simulink model "mainModel"  (R2018b)
settings: Solver=ode15s  StartTime=0.0  StopTime=sim_time  MaxStep=maxStep* tp.lengthScaleFactor^0.5
values from neighbouring files (symbols this model uses):
  grav = 9.81    [mainModel_ts.m]
  MI = [14330000 0 0; 0 143200 0; 0 0 15300000]    [mainModel_ts.m]
undefined symbols (not defined in the file or in its folder): env_t, tp
libraries: tethersNCsContrl_cl x1, fixedGroundStation_cl x1, avl2DLiftingBdy_cl x1, partitionedLifitngBdy_cls x1, kelvinVoigtTether_cl x1, pureIntegratorWinch_cl x1
settings Model: SimulationMode=accelerator  Creator=Ayaz  LastModifiedBy=asiddiq2

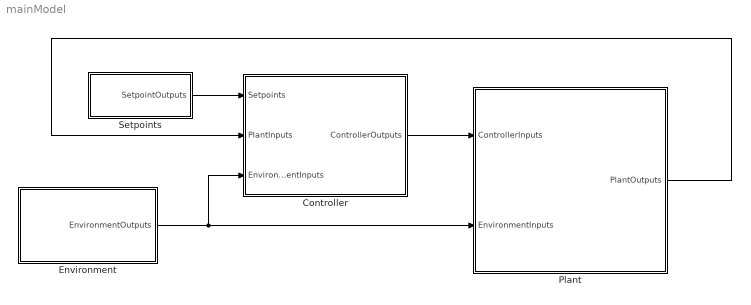
== system mainModel ==
  Controller : Subsystem
  Environment : Subsystem
  Plant : Subsystem
  Setpoints : Subsystem
  wires:
  Environment/1(EnvironmentOutputs) -> Plant/2(EnvironmentInputs), Controller/3(EnvironmentInputs)
  Plant/1(PlantOutputs) -> Controller/2(PlantInputs)
  Controller/1(ControllerOutputs) -> Plant/1(ControllerInputs)
  Setpoints/1(SetpointOutputs) -> Controller/1(Setpoints)

== system mainModel/Controller ==
  Setpoints : Inport
  PlantInputs : Inport  Port=2
  EnvironmentInputs : Inport  Port=3
  Variant Subsystem : Subsystem  VariantControlMode=Label  Variant=on  LabelModeActiveChoice=tethersNCsVariant  mask{ctlr_var=Simple Tether and Control Surfaces}
      mask prompts: ctlr_var "Choose Controller Variant"
      mask init:
      | choice = get_param(gcb,'ctlr_var');
      | vssBlk = gcb;
      | 
      | if strcmp(choice,'Simple Tether and Control Surfaces')
      |     set_param(vssBlk, 'OverrideUsingVariant', 'tethersNCsVariant');
      |     
      | elseif strcmp(choice,'No Controller')
      |     set_param(vssBlk, 'OverrideUsingVariant', 'NoControl');
      |     
      | end
      mask TypeOptions ctlr_var: Simple Tether and Control Surfaces | No Controller
  ControllerOutputs : Outport
  wires:
  EnvironmentInputs/1 -> Variant Subsystem/3(EnvironmentOutputs)
  PlantInputs/1 -> Variant Subsystem/2(PlantOutputs)
  Setpoints/1 -> Variant Subsystem/1(Setpoints)
  Variant Subsystem/1(ControllerOutputs) -> ControllerOutputs/1

== system mainModel/Environment ==
  Bus Creator : BusCreator  Inputs=1
  Constant : Constant  Value=env_t.inertialFlowVel.value  VectorParams1D=off
  Reshape : Reshape  OutputDimensionality=Column vector (2-D)
  EnvironmentOutputs : Outport
  wires:
  Constant/1 -> Reshape/1
  Reshape/1 -> Bus Creator/1  "inertialFlowVel"
  Bus Creator/1 -> EnvironmentOutputs/1

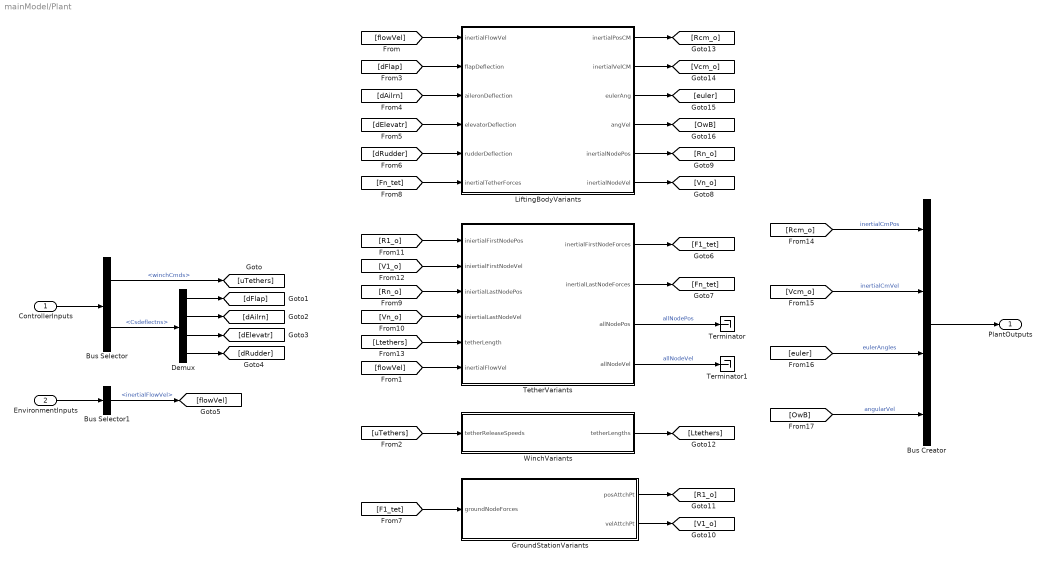
== system mainModel/Plant ==
  ControllerInputs : Inport
  EnvironmentInputs : Inport  Port=2
  Bus Creator : BusCreator  Inputs=4
  Bus Selector : BusSelector  OutputSignals=winchCmds,Csdeflectns
  Bus Selector1 : BusSelector  OutputSignals=inertialFlowVel
  Demux : Demux
  GroundStationVariants : Subsystem  VariantControlMode=Label  Variant=on  LabelModeActiveChoice=FixedVariant  mask{gndStatnMdl=Fixed Ground Station}
      mask prompts: gndStatnMdl "Choose Ground Station Model"
      mask init:
      | choice = get_param(gcb,'gndStatnMdl');
      | vssBlk = gcb;
      | 
      | if strcmp(choice,'Fixed Ground Station')
      |     set_param(vssBlk, 'OverrideUsingVariant', 'FixedVariant');
      |     
      | elseif strcmp(choice,'Floating Ground Station')
      |     set_param(vssBlk, 'OverrideUsingVariant', 'FloatingVariant');
      |     
      | end
      mask TypeOptions gndStatnMdl: Fixed Ground Station | Floating Ground Station
  LiftingBodyVariants : Subsystem  VariantControlMode=Label  Variant=on  LabelModeActiveChoice=partitionedLftingBdyVariant  mask{lftingbdyMdl=Partitioned Lifting Body}
      mask prompts: lftingbdyMdl "Choose Lifting Body Model"
      mask init:
      | choice = get_param(gcb,'lftingbdyMdl');
      | vssBlk = gcb;
      | 
      | if strcmp(choice,'AVL 2D Lifting Body')
      |     set_param(vssBlk, 'OverrideUsingVariant', 'AVL2dVariant');
      |     
      | elseif strcmp(choice,'Ayaz OCT Lifitng Body')
      |     set_param(vssBlk, 'OverrideUsingVariant', 'AyazOctVariant');
      |     
      | elseif strcmp(choice,'Partitioned Lifting Body')
      |     set_param(vssBlk, 'OverrideUsingVariant', 'partitionedLftingBdyVariant');
      |     
      | end
      mask TypeOptions lftingbdyMdl: AVL 2D Lifting Body | Ayaz OCT Lifitng Body | Partitioned Lifting Body
  Terminator : Terminator
  Terminator1 : Terminator
  TetherVariants : Subsystem  VariantControlMode=Label  Variant=on  LabelModeActiveChoice=KelvinVoigtVariant  mask{tetherMdl=Kelvin Voigt Model}
      mask prompts: tetherMdl "Choose Tether Model"
      mask init:
      | choice = get_param(gcb,'tetherMdl');
      | vssBlk = gcb;
      | 
      | if strcmp(choice,'Kelvin Voigt Model')
      |     set_param(vssBlk, 'OverrideUsingVariant', 'KelvinVoigtVariant');
      |     
      | elseif strcmp(choice,'No Model')
      |     set_param(vssBlk, 'OverrideUsingVariant', 'NoTetherVariant');
      |     
      | end
      mask TypeOptions tetherMdl: Kelvin Voigt Model | No Model
  WinchVariants : Subsystem  VariantControlMode=Label  Variant=on  LabelModeActiveChoice=PureIntegratorVariant  mask{winchMdl=Pure Integrator Winch}
      mask prompts: winchMdl "Choose Winch Model"
      mask init:
      | choice = get_param(gcb,'winchMdl');
      | vssBlk = gcb;
      | 
      | if strcmp(choice,'Pure Integrator Winch')
      |     set_param(vssBlk, 'OverrideUsingVariant', 'PureIntegratorVariant');
      |     
      | elseif strcmp(choice,'No Winch')
      |     set_param(vssBlk, 'OverrideUsingVariant', 'NoWinchVariant');
      |     
      | end
      mask TypeOptions winchMdl: Pure Integrator Winch | No Winch
  PlantOutputs : Outport
  wires:
  [OwB] -> Bus Creator/4  "angularVel"
  [euler] -> Bus Creator/3  "eulerAngles"
  [Vcm_o] -> Bus Creator/2  "inertialCmVel"
  [Rcm_o] -> Bus Creator/1  "inertialCmPos"
  Bus Creator/1 -> PlantOutputs/1
  ControllerInputs/1 -> Bus Selector/1
  Bus Selector/1 -> [uTethers]  "<winchCmds>"
  [flowVel] -> LiftingBodyVariants/1(inertialFlowVel)
  [uTethers] -> WinchVariants/1(tetherReleaseSpeeds)
  [dFlap] -> LiftingBodyVariants/2(flapDeflection)
  [dRudder] -> LiftingBodyVariants/5(rudderDeflection)
  [dElevatr] -> LiftingBodyVariants/4(elevatorDeflection)
  [dAilrn] -> LiftingBodyVariants/3(aileronDeflection)
  TetherVariants/1(inertialFirstNodeForces) -> [F1_tet]
  [F1_tet] -> GroundStationVariants/1(groundNodeForces)
  TetherVariants/2(inertialLastNodeForces) -> [Fn_tet]
  [Fn_tet] -> LiftingBodyVariants/6(inertialTetherForces)
  LiftingBodyVariants/6(inertialNodeVel) -> [Vn_o]
  LiftingBodyVariants/5(inertialNodePos) -> [Rn_o]
  [Vn_o] -> TetherVariants/4(iniertialLastNodeVel)
  [Rn_o] -> TetherVariants/3(iniertialLastNodePos)
  GroundStationVariants/1(posAttchPt) -> [R1_o]
  GroundStationVariants/2(velAttchPt) -> [V1_o]
  [R1_o] -> TetherVariants/1(iniertialFirstNodePos)
  [V1_o] -> TetherVariants/2(iniertialFirstNodeVel)
  TetherVariants/3(allNodePos) -> Terminator/1  "allNodePos"
  TetherVariants/4(allNodeVel) -> Terminator1/1  "allNodeVel"
  LiftingBodyVariants/1(inertialPosCM) -> [Rcm_o]
  LiftingBodyVariants/2(inertialVelCM) -> [Vcm_o]
  LiftingBodyVariants/3(eulerAng) -> [euler]
  LiftingBodyVariants/4(angVel) -> [OwB]
  [Ltethers] -> TetherVariants/5(tetherLength)
  [flowVel] -> TetherVariants/6(inertialFlowVel)
  WinchVariants/1(tetherLengths) -> [Ltethers]
  EnvironmentInputs/1 -> Bus Selector1/1
  Bus Selector1/1 -> [flowVel]  "<inertialFlowVel>"
  Bus Selector/2 -> Demux/1  "<Csdeflectns>"
  Demux/1 -> [dFlap]
  Demux/2 -> [dAilrn]
  Demux/3 -> [dElevatr]
  Demux/4 -> [dRudder]

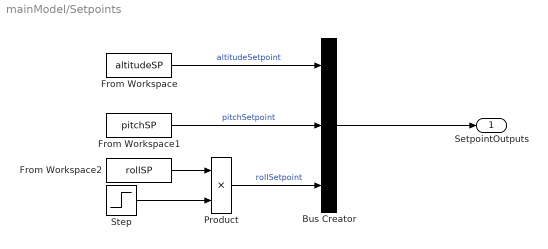
== system mainModel/Setpoints ==
  Bus Creator : BusCreator  Inputs=3
  From Workspace : FromWorkspace  VariableName=altitudeSP  SampleTime=0
  From Workspace1 : FromWorkspace  VariableName=pitchSP  SampleTime=0
  From Workspace2 : FromWorkspace  VariableName=rollSP  SampleTime=0
  Product : Product
  Step : Step  Time=30*sqrt(tp.lengthScaleFactor)  SampleTime=0
  SetpointOutputs : Outport
  wires:
  Bus Creator/1 -> SetpointOutputs/1
  Product/1 -> Bus Creator/3  "rollSetpoint"
  From Workspace1/1 -> Bus Creator/2  "pitchSetpoint"
  From Workspace/1 -> Bus Creator/1  "altitudeSetpoint"
  From Workspace2/1 -> Product/1
  Step/1 -> Product/2

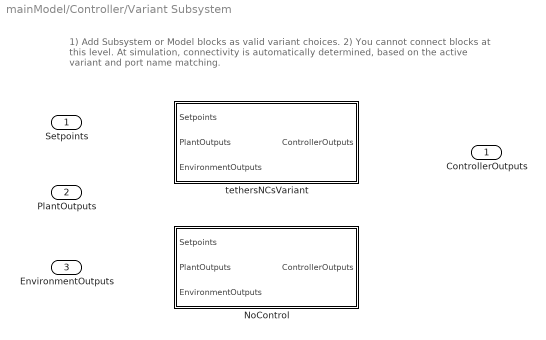
== system mainModel/Controller/Variant Subsystem ==
  note: 1) Add Subsystem or Model blocks as valid variant choices.
      | 2) You cannot connect blocks at this level. At simulation, connectivity is automatically
      | determined, based on the active variant and port name matching.
  Setpoints : Inport
  PlantOutputs : Inport  Port=2
  EnvironmentOutputs : Inport  Port=3
  NoControl : Subsystem  VariantControl=NoControl
  tethersNCsVariant : Subsystem  VariantControl=tethersNCsVariant
  ControllerOutputs : Outport

== system mainModel/Plant/GroundStationVariants ==
  note: 1) Add Subsystem or Model blocks as valid variant choices.
      | 2) You cannot connect blocks at this level. At simulation, connectivity is automatically
      | determined, based on the active variant and port name matching.
  groundNodeForces : Inport
  FixedVariant : Subsystem  VariantControl=FixedVariant
  FloatingVariant : Subsystem  VariantControl=FloatingVariant
  posAttchPt : Outport
  velAttchPt : Outport  Port=2

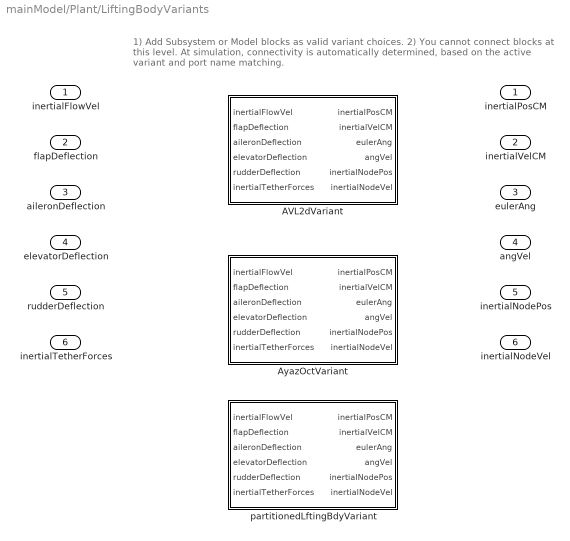
== system mainModel/Plant/LiftingBodyVariants ==
  note: 1) Add Subsystem or Model blocks as valid variant choices.
      | 2) You cannot connect blocks at this level. At simulation, connectivity is automatically
      | determined, based on the active variant and port name matching.
  inertialFlowVel : Inport
  flapDeflection : Inport  Port=2
  aileronDeflection : Inport  Port=3
  elevatorDeflection : Inport  Port=4
  rudderDeflection : Inport  Port=5
  inertialTetherForces : Inport  Port=6
  AVL2dVariant : Subsystem  VariantControl=AVL2dVariant
  AyazOctVariant : Subsystem  VariantControl=AyazOctVariant
  partitionedLftingBdyVariant : Subsystem  VariantControl=partitionedLftingBdyVariant
  inertialPosCM : Outport
  inertialVelCM : Outport  Port=2
  eulerAng : Outport  Port=3
  angVel : Outport  Port=4
  inertialNodePos : Outport  Port=5
  inertialNodeVel : Outport  Port=6

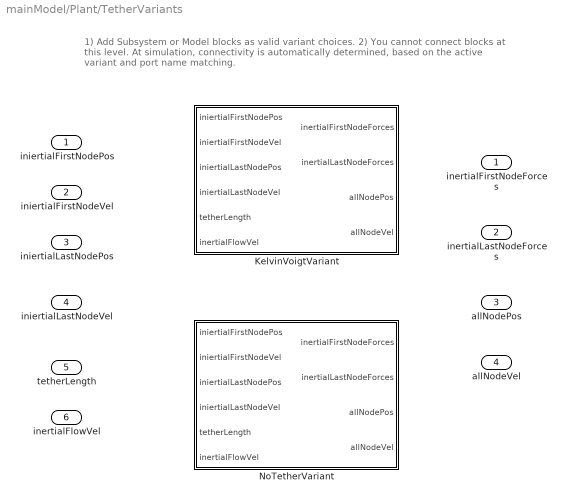
== system mainModel/Plant/TetherVariants ==
  note: 1) Add Subsystem or Model blocks as valid variant choices.
      | 2) You cannot connect blocks at this level. At simulation, connectivity is automatically
      | determined, based on the active variant and port name matching.
  iniertialFirstNodePos : Inport
  iniertialFirstNodeVel : Inport  Port=2
  iniertialLastNodePos : Inport  Port=3
  iniertialLastNodeVel : Inport  Port=4
  tetherLength : Inport  Port=5
  inertialFlowVel : Inport  Port=6
  KelvinVoigtVariant : Subsystem  VariantControl=KelvinVoigtVariant
  NoTetherVariant : Subsystem  VariantControl=NoTetherVariant
  inertialFirstNodeForces : Outport
  inertialLastNodeForces : Outport  Port=2
  allNodePos : Outport  Port=3
  allNodeVel : Outport  Port=4

== system mainModel/Plant/WinchVariants ==
  note: 1) Add Subsystem or Model blocks as valid variant choices.
      | 2) You cannot connect blocks at this level. At simulation, connectivity is automatically
      | determined, based on the active variant and port name matching.
  tetherReleaseSpeeds : Inport
  NoWinchVariant : Subsystem  VariantControl=NoWinchVariant
  PureIntegratorVariant : Subsystem  VariantControl=PureIntegratorVariant
  tetherLengths : Outport

== system mainModel/Controller/Variant Subsystem/NoControl ==
  Setpoints : Inport
  PlantOutputs : Inport  Port=2
  EnvironmentOutputs : Inport  Port=3
  ControllerOutputs : Outport

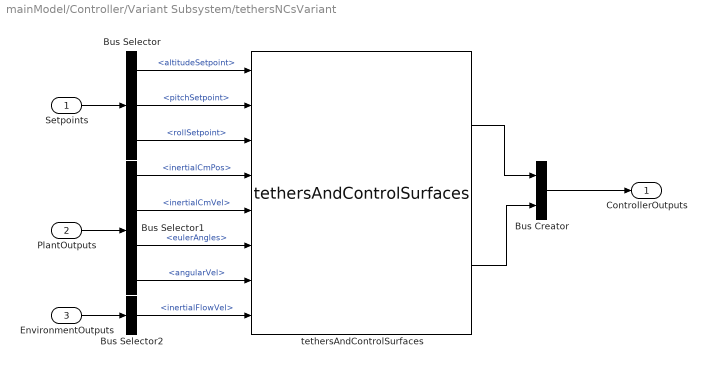
== system mainModel/Controller/Variant Subsystem/tethersNCsVariant ==
  Setpoints : Inport
  PlantOutputs : Inport  Port=2
  EnvironmentOutputs : Inport  Port=3
  Bus Creator : BusCreator  Inputs=2
  Bus Selector : BusSelector  OutputSignals=altitudeSetpoint,pitchSetpoint,rollSetpoint
  Bus Selector1 : BusSelector  OutputSignals=inertialCmPos,inertialCmVel,eulerAngles,angularVel
  Bus Selector2 : BusSelector  OutputSignals=inertialFlowVel
  tethersAndControlSurfaces : tethersNCsContrl_cl/tethersAndControlSurfaces  thr_clr=ctrllr.tethers  cs_clr=ctrllr.controlSurfaces
  ControllerOutputs : Outport
  wires:
  Setpoints/1 -> Bus Selector/1
  Bus Selector/1 -> tethersAndControlSurfaces/1  "<altitudeSetpoint>"
  Bus Selector/2 -> tethersAndControlSurfaces/2  "<pitchSetpoint>"
  Bus Selector/3 -> tethersAndControlSurfaces/3  "<rollSetpoint>"
  PlantOutputs/1 -> Bus Selector1/1
  Bus Selector1/1 -> tethersAndControlSurfaces/4  "<inertialCmPos>"
  Bus Selector1/2 -> tethersAndControlSurfaces/5  "<inertialCmVel>"
  Bus Selector1/3 -> tethersAndControlSurfaces/6  "<eulerAngles>"
  Bus Selector1/4 -> tethersAndControlSurfaces/7  "<angularVel>"
  EnvironmentOutputs/1 -> Bus Selector2/1
  Bus Selector2/1 -> tethersAndControlSurfaces/8  "<inertialFlowVel>"
  tethersAndControlSurfaces/1 -> Bus Creator/1
  tethersAndControlSurfaces/2 -> Bus Creator/2
  Bus Creator/1 -> ControllerOutputs/1

== system mainModel/Plant/GroundStationVariants/FixedVariant ==
  groundNodeForces : Inport
  fixedGroundStation : fixedGroundStation_cl/fixedGroundStation  gs_switch=tp.gndStation.rotationSwitch.value  Izz=tp.gndStation.Izz.value  plat_damp_coeff=tp.gndStation.dampCoeff.value  ini_psiPlat=tp.gndStation.ini_platform_ang.value  ini_OwP=tp.gndStation.ini_platform_vel.value  attchPtSturct=tp.gndStationTetherAttchPts
  posAttchPt : Outport
  velAttchPt : Outport  Port=2
  wires:
  groundNodeForces/1 -> fixedGroundStation/1
  fixedGroundStation/1 -> posAttchPt/1
  fixedGroundStation/2 -> velAttchPt/1

== system mainModel/Plant/GroundStationVariants/FloatingVariant ==
  groundNodeForces : Inport
  Zero : Constant  Value=0  OutDataTypeStr=Inherit: Inherit via back propagation
  posAttchPt : Outport
  velAttchPt : Outport  Port=2
  wires:
  Zero/1 -> velAttchPt/1
  groundNodeForces/1 -> posAttchPt/1

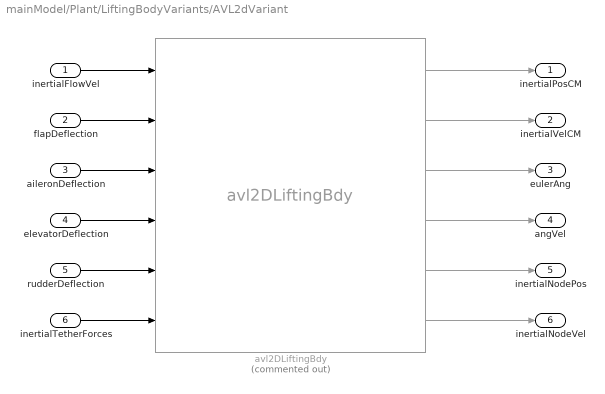
== system mainModel/Plant/LiftingBodyVariants/AVL2dVariant ==
  inertialFlowVel : Inport
  flapDeflection : Inport  Port=2
  aileronDeflection : Inport  Port=3
  elevatorDeflection : Inport  Port=4
  rudderDeflection : Inport  Port=5
  inertialTetherForces : Inport  Port=6
  avl2DLiftingBdy : avl2DLiftingBdy_cl/avl2DLiftingBdy  Commented=on  M=mass  M_added=m_added  J=MI  vol=vol  Rcb_cm=Rcb_cm  turb_struct=turbine  cls_obj=class_liftingBdy  g=grav  rho_fluid=rho_fluid  initPos=ini_Rcm_o  initVel=ini_O_Vcm_o  initEulAngs=ini_euler  initAngVel=ini_OwB  CLTable=CLtot_2D_Tbl  CDTable=CDtot_2D_Tbl  CMxTable=Cltot_2D_Tbl  CMyTable=Cmtot_2D_Tbl  CMzTable=Cntot_2D_Tbl  CsGainMatrix=k_CS_gain  CRef=Cref  BRef=Bref  SRef=Sref
  inertialPosCM : Outport
  inertialVelCM : Outport  Port=2
  eulerAng : Outport  Port=3
  angVel : Outport  Port=4
  inertialNodePos : Outport  Port=5
  inertialNodeVel : Outport  Port=6
  wires:
  rudderDeflection/1 -> avl2DLiftingBdy/5
  inertialTetherForces/1 -> avl2DLiftingBdy/6
  flapDeflection/1 -> avl2DLiftingBdy/2
  elevatorDeflection/1 -> avl2DLiftingBdy/4
  aileronDeflection/1 -> avl2DLiftingBdy/3
  inertialFlowVel/1 -> avl2DLiftingBdy/1
  avl2DLiftingBdy/6 -> inertialNodeVel/1
  avl2DLiftingBdy/4 -> angVel/1
  avl2DLiftingBdy/3 -> eulerAng/1
  avl2DLiftingBdy/5 -> inertialNodePos/1
  avl2DLiftingBdy/1 -> inertialPosCM/1
  avl2DLiftingBdy/2 -> inertialVelCM/1

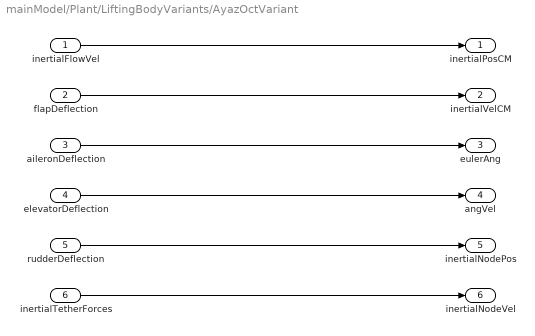
== system mainModel/Plant/LiftingBodyVariants/AyazOctVariant ==
  inertialFlowVel : Inport
  flapDeflection : Inport  Port=2
  aileronDeflection : Inport  Port=3
  elevatorDeflection : Inport  Port=4
  rudderDeflection : Inport  Port=5
  inertialTetherForces : Inport  Port=6
  inertialPosCM : Outport
  inertialVelCM : Outport  Port=2
  eulerAng : Outport  Port=3
  angVel : Outport  Port=4
  inertialNodePos : Outport  Port=5
  inertialNodeVel : Outport  Port=6
  wires:
  rudderDeflection/1 -> inertialNodePos/1
  elevatorDeflection/1 -> angVel/1
  flapDeflection/1 -> inertialVelCM/1
  inertialFlowVel/1 -> inertialPosCM/1
  inertialTetherForces/1 -> inertialNodeVel/1
  aileronDeflection/1 -> eulerAng/1

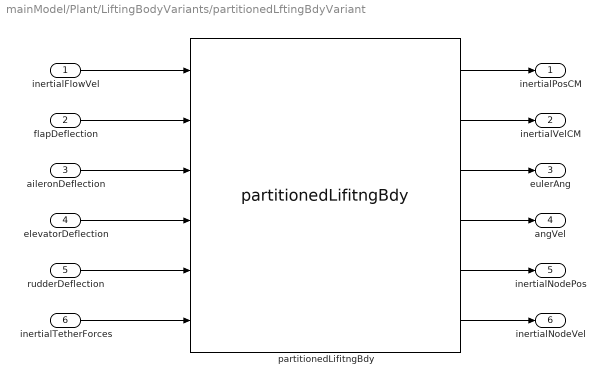
== system mainModel/Plant/LiftingBodyVariants/partitionedLftingBdyVariant ==
  inertialFlowVel : Inport
  flapDeflection : Inport  Port=2
  aileronDeflection : Inport  Port=3
  elevatorDeflection : Inport  Port=4
  rudderDeflection : Inport  Port=5
  inertialTetherForces : Inport  Port=6
  partitionedLifitngBdy : partitionedLifitngBdy_cls/partitionedLifitngBdy  massBdy=tp.vehicle.mass.value  massAdded=tp.vehicle.added_mass.value  miBdy=tp.vehicle.MI.value  volBdy=tp.vehicle.volume.value  Rcb_cm=tp.vehicle.Rcb_cm.value  turbStruct=tp.turbines  attchPtSturct=tp.vehicleTetherAttchPts  gravAcc=env_t.gravAccel.value  rhoFluid=env_t.flowDensity.value  aero_struct=tp.aeroCoeffData  initPos=tp.vehicle.ini_Rcm_o.value  initVel=tp.vehicle.ini_O_Vcm_o.value  initEulAngs=tp.vehicle.ini_euler.value  initAngVel=tp.vehicle.ini_OwB.value
  inertialPosCM : Outport
  inertialVelCM : Outport  Port=2
  eulerAng : Outport  Port=3
  angVel : Outport  Port=4
  inertialNodePos : Outport  Port=5
  inertialNodeVel : Outport  Port=6
  wires:
  elevatorDeflection/1 -> partitionedLifitngBdy/4
  rudderDeflection/1 -> partitionedLifitngBdy/5
  aileronDeflection/1 -> partitionedLifitngBdy/3
  inertialTetherForces/1 -> partitionedLifitngBdy/6
  flapDeflection/1 -> partitionedLifitngBdy/2
  inertialFlowVel/1 -> partitionedLifitngBdy/1
  partitionedLifitngBdy/1 -> inertialPosCM/1
  partitionedLifitngBdy/3 -> eulerAng/1
  partitionedLifitngBdy/4 -> angVel/1
  partitionedLifitngBdy/2 -> inertialVelCM/1
  partitionedLifitngBdy/6 -> inertialNodeVel/1
  partitionedLifitngBdy/5 -> inertialNodePos/1

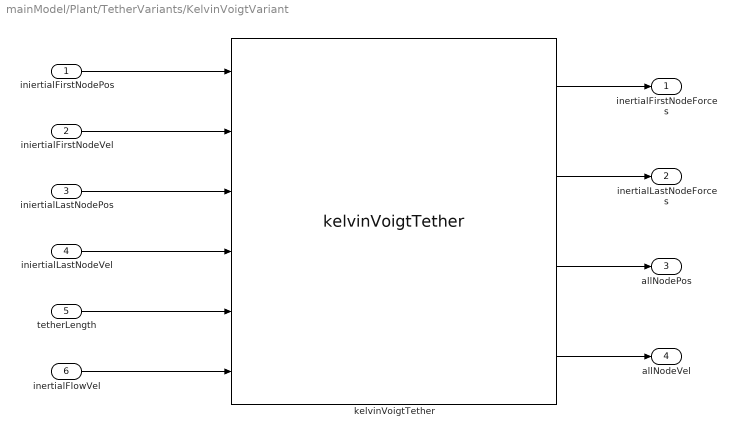
== system mainModel/Plant/TetherVariants/KelvinVoigtVariant ==
  iniertialFirstNodePos : Inport
  iniertialFirstNodeVel : Inport  Port=2
  iniertialLastNodePos : Inport  Port=3
  iniertialLastNodeVel : Inport  Port=4
  tetherLength : Inport  Port=5
  inertialFlowVel : Inport  Port=6
  kelvinVoigtTether : kelvinVoigtTether_cl/kelvinVoigtTether  LabelModeActiveChoice=tetherNumNode2Variant  KVmodel=2 node model  rhoFluid=env_t.flowDensity.value  gravAccl=env_t.gravAccel.value  massBdy=tp.vehicle.mass.value  numNode=[tp.tethers.numNodes]  diaTether=[tp.tethers.diameter]  rhoTether=[tp.tethers.density]  youngsTether=[tp.tethers.youngsModulus]  zetaTether=[tp.tethers.dampingRatio]  CdTether=[tp.tethers.dragCoeff]
  inertialFirstNodeForces : Outport
  inertialLastNodeForces : Outport  Port=2
  allNodePos : Outport  Port=3
  allNodeVel : Outport  Port=4
  wires:
  iniertialLastNodePos/1 -> kelvinVoigtTether/3
  iniertialLastNodeVel/1 -> kelvinVoigtTether/4
  iniertialFirstNodeVel/1 -> kelvinVoigtTether/2
  iniertialFirstNodePos/1 -> kelvinVoigtTether/1
  kelvinVoigtTether/3 -> allNodePos/1
  kelvinVoigtTether/4 -> allNodeVel/1
  kelvinVoigtTether/2 -> inertialLastNodeForces/1
  kelvinVoigtTether/1 -> inertialFirstNodeForces/1
  inertialFlowVel/1 -> kelvinVoigtTether/6
  tetherLength/1 -> kelvinVoigtTether/5

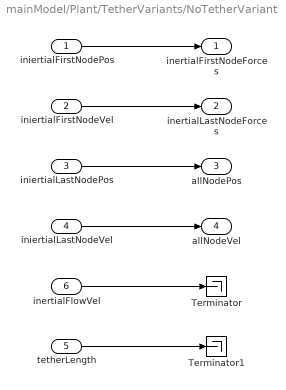
== system mainModel/Plant/TetherVariants/NoTetherVariant ==
  iniertialFirstNodePos : Inport
  iniertialFirstNodeVel : Inport  Port=2
  iniertialLastNodePos : Inport  Port=3
  iniertialLastNodeVel : Inport  Port=4
  tetherLength : Inport  Port=5
  inertialFlowVel : Inport  Port=6
  Terminator : Terminator
  Terminator1 : Terminator
  inertialFirstNodeForces : Outport
  inertialLastNodeForces : Outport  Port=2
  allNodePos : Outport  Port=3
  allNodeVel : Outport  Port=4
  wires:
  tetherLength/1 -> Terminator1/1
  iniertialFirstNodeVel/1 -> inertialLastNodeForces/1
  inertialFlowVel/1 -> Terminator/1
  iniertialFirstNodePos/1 -> inertialFirstNodeForces/1
  iniertialLastNodeVel/1 -> allNodeVel/1
  iniertialLastNodePos/1 -> allNodePos/1

== system mainModel/Plant/WinchVariants/NoWinchVariant ==
  tetherReleaseSpeeds : Inport
  tetherLengths : Outport

== system mainModel/Plant/WinchVariants/PureIntegratorVariant ==
  tetherReleaseSpeeds : Inport
  PureIntegratorWinch : pureIntegratorWinch_cl/PureIntegratorWinch  u_max=[tp.winches.maxSpeed]  wTau=[tp.winches.timeConstant]  iniTetL=[tp.winches.initTetherLength]
  Reshape : Reshape  OutputDimensionality=Column vector (2-D)
  Terminator : Terminator
  tetherLengths : Outport
  wires:
  tetherReleaseSpeeds/1 -> PureIntegratorWinch/1
  PureIntegratorWinch/1 -> tetherLengths/1
  Reshape/1 -> Terminator/1  "thrReleseSpeeds"
  PureIntegratorWinch/2 -> Reshape/1
